simulink model "chap8_2sim"  (Simulink 3.00)
settings: Solver=ode45  StartTime=0.0  StopTime=5  RelTol=1e-3
settings Model: LastModifiedBy=liu

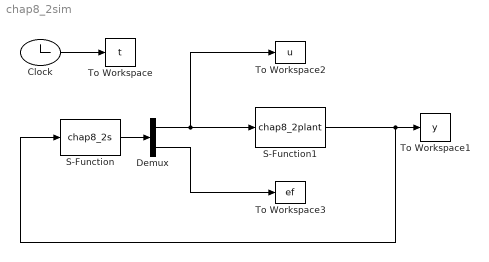
== system chap8_2sim ==
  Clock : Clock
  Demux : Demux  Outputs=2
  S-Function : S-Function  FunctionName=chap8_2s  PortCounts=[]  SFunctionModules=''
  S-Function1 : S-Function  FunctionName=chap8_2plant  PortCounts=[]  SFunctionModules=''
  To Workspace : ToWorkspace  VariableName=t  SampleTime=-1  SaveFormat=Matrix
  To Workspace1 : ToWorkspace  VariableName=y  SampleTime=-1  SaveFormat=Matrix
  To Workspace2 : ToWorkspace  VariableName=u  SampleTime=-1  SaveFormat=Matrix
  To Workspace3 : ToWorkspace  VariableName=ef  SampleTime=-1  SaveFormat=Matrix
  wires:
  S-Function/1 -> Demux/1
  Demux/1 -> S-Function1/1, To Workspace2/1
  Demux/2 -> To Workspace3/1
  Clock/1 -> To Workspace/1
  S-Function1/1 -> To Workspace1/1, S-Function/1
